simulink model "sim_topic4"  (R2023b)
settings: Solver=FixedStepAuto  StartTime=0.0  StopTime=T_sim  FixedStep=dt_sim  RelTol=1e-3
undefined symbols (not defined in the file): den_Gd1_tf, den_Gd2_tf, num_Gd1_tf, num_Gd2_tf, T
settings Model: Creator=user  LastModifiedBy=user

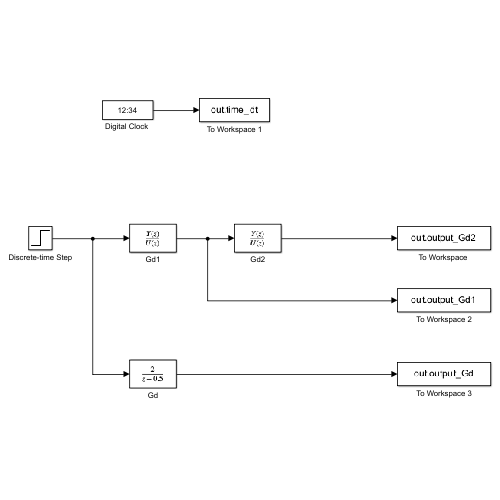
[thumbnail: Simulink's stored preview of the top-level diagram]
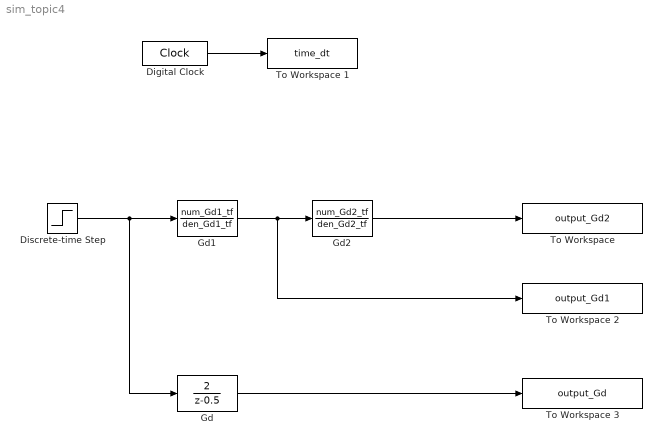
== system sim_topic4 ==
  "Digital Clock " : DigitalClock  SampleTime=T
  Discrete-time Step : Step  Time=0  SampleTime=T
  Gd : DiscreteTransferFcn  Numerator=2  Denominator=[1 -0.5]
  Gd1 : DiscreteTransferFcn  Numerator=num_Gd1_tf  Denominator=den_Gd1_tf
  Gd2 : DiscreteTransferFcn  Numerator=num_Gd2_tf  Denominator=den_Gd2_tf
  "To Workspace " : ToWorkspace  VariableName=output_Gd2  SampleTime=T
  To Workspace 1 : ToWorkspace  VariableName=time_dt  SampleTime=T
  To Workspace 2 : ToWorkspace  VariableName=output_Gd1  SampleTime=T
  To Workspace 3 : ToWorkspace  VariableName=output_Gd  SampleTime=T
  wires:
  "Digital Clock "/1 -> To Workspace 1/1
  Gd2/1 -> "To Workspace "/1
  Discrete-time Step/1 -> Gd/1, Gd1/1
  Gd1/1 -> To Workspace 2/1, Gd2/1
  Gd/1 -> To Workspace 3/1
